simulink model "DinamicaCinematicaOrbital"  (R2024a)
settings: Solver=FixedStepAuto  StartTime=0.0  StopTime=tf  FixedStep=step_modelo  RelTol=1e-8  AbsTol=abs_tol
values from neighbouring files (symbols this model uses):
  J2 = 1082.63E-6    (= 0.00108263)    [constantes.m]
  mi = 3.9860044189*10^14    (= 398600441890000)    [constantes.m]
  omega_E = 7.29211585530*10^-5    (= 7.2921158553e-05)    [constantes.m]
  Re = 6378.1363*10^3    (= 6378136.3)    [constantes.m]
undefined symbols (not defined in the file or in its folder): a0_ini, Cd0, Cd1, drag, e0_ini, f0_ini, i0_ini, J2_dist, L0, L1, m0, m1, ohm0_ini, omega0_ini, pcoRad, r0, r0_dot_ini, t_man, theta0_ini, x0_dot, x0_dot_i, x0_dot_ini, x0_i, x0_ini, y0_dot_i, y0_dot_ini, y0_i, y0_ini, z0_dot_i, z0_dot_ini, z0_i, z0_ini
libraries: simulink x5
settings Model: PacingRate=500  Creator=rodri  LastModifiedBy=rodri
settings DataIOCC: SaveOutput=off  SaveTime=off
settings ModelReferenceCC: EnableRefExpFcnMdlSchedulingChecks=on
settings RTWCC: GPUComputeCapability=3.5

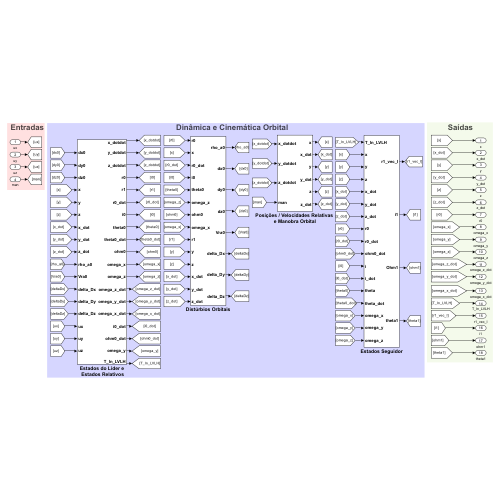
[thumbnail: Simulink's stored preview of the top-level diagram]
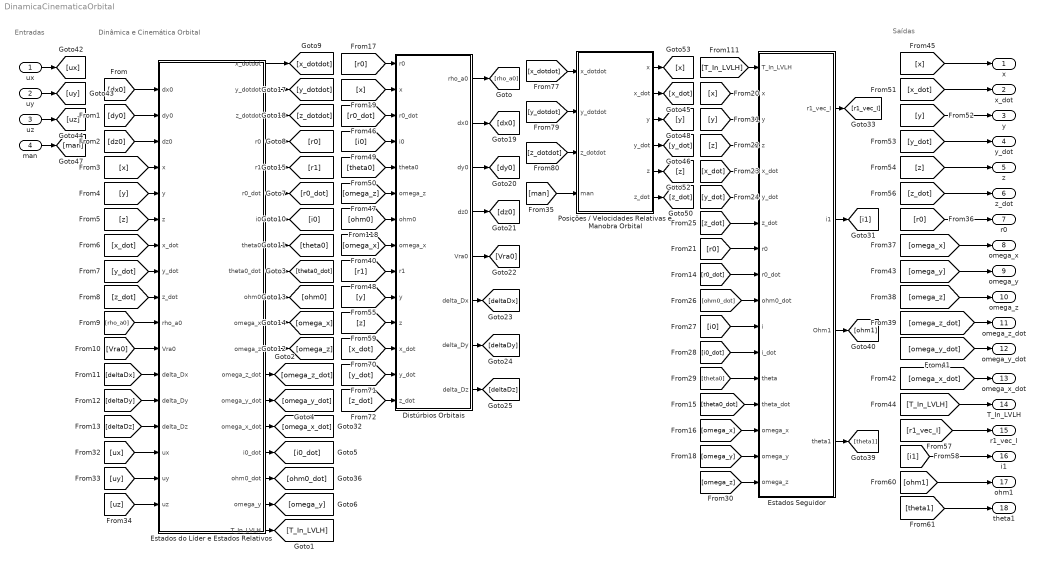
== system DinamicaCinematicaOrbital ==
  note: Saídas
  note: Dinâmica e Cinemática Orbital
  note: Entradas
  ux : Inport  OutDataTypeStr=double  PortDimensions=1
  uy : Inport  Port=2  OutDataTypeStr=double  PortDimensions=1
  uz : Inport  Port=3  OutDataTypeStr=double  PortDimensions=1
  man : Inport  Port=4  OutDataTypeStr=boolean
  Distúrbios Orbitais : Subsystem
  Estados Seguidor : Subsystem
  Estados do Líder e Estados Relativos : Subsystem
  Posições / Velocidades Relativas e Manobra Orbital : Subsystem
  x : Outport  OutDataTypeStr=double  PortDimensions=1  SampleTime=0
  x_dot : Outport  Port=2  OutDataTypeStr=double  PortDimensions=1  SampleTime=0
  y : Outport  Port=3  OutDataTypeStr=double  PortDimensions=1  SampleTime=0
  y_dot : Outport  Port=4  OutDataTypeStr=double  PortDimensions=1  SampleTime=0
  z : Outport  Port=5  OutDataTypeStr=double  PortDimensions=1  SampleTime=0
  z_dot : Outport  Port=6  OutDataTypeStr=double  PortDimensions=1  SampleTime=0
  r0 : Outport  Port=7  OutDataTypeStr=double  PortDimensions=1  SampleTime=0
  omega_x : Outport  Port=8  OutDataTypeStr=double  PortDimensions=1  SampleTime=0
  omega_y : Outport  Port=9
  omega_z : Outport  Port=10  OutDataTypeStr=double  PortDimensions=1  SampleTime=0
  omega_z_dot : Outport  Port=11  OutDataTypeStr=double  PortDimensions=1  SampleTime=0
  omega_y_dot : Outport  Port=12  OutDataTypeStr=double  PortDimensions=1  SampleTime=0
  omega_x_dot : Outport  Port=13  OutDataTypeStr=double  PortDimensions=1  SampleTime=0
  T_In_LVLH : Outport  Port=14
  r1_vec_I : Outport  Port=15
  i1 : Outport  Port=16
  ohm1 : Outport  Port=17
  theta1 : Outport  Port=18
  wires:
  Posições / Velocidades Relativas e Manobra Orbital/5(z) -> [z]
  Posições / Velocidades Relativas e Manobra Orbital/2(x_dot) -> [x_dot]
  Posições / Velocidades Relativas e Manobra Orbital/4(y_dot) -> [y_dot]
  Posições / Velocidades Relativas e Manobra Orbital/6(z_dot) -> [z_dot]
  Posições / Velocidades Relativas e Manobra Orbital/3(y) -> [y]
  Posições / Velocidades Relativas e Manobra Orbital/1(x) -> [x]
  Distúrbios Orbitais/1(rho_a0) -> [rho_a0]
  Estados do Líder e Estados Relativos/18(omega_y) -> [omega_y]
  Estados do Líder e Estados Relativos/14(omega_y_dot) -> [omega_y_dot]
  Estados do Líder e Estados Relativos/19(T_In_LVLH) -> [T_In_LVLH]
  Estados do Líder e Estados Relativos/13(omega_z_dot) -> [omega_z_dot]
  Estados do Líder e Estados Relativos/16(i0_dot) -> [i0_dot]
  Estados do Líder e Estados Relativos/12(omega_z) -> [omega_z]
  Estados do Líder e Estados Relativos/10(ohm0) -> [ohm0]
  Estados do Líder e Estados Relativos/2(y_dotdot) -> [y_dotdot]
  Estados do Líder e Estados Relativos/11(omega_x) -> [omega_x]
  Estados do Líder e Estados Relativos/4(r0) -> [r0]
  Estados do Líder e Estados Relativos/3(z_dotdot) -> [z_dotdot]
  Estados do Líder e Estados Relativos/6(r0_dot) -> [r0_dot]
  Estados do Líder e Estados Relativos/1(x_dotdot) -> [x_dotdot]
  Estados do Líder e Estados Relativos/8(theta0) -> [theta0]
  Estados do Líder e Estados Relativos/5(r1) -> [r1]
  Estados do Líder e Estados Relativos/7(i0) -> [i0]
  Estados do Líder e Estados Relativos/17(ohm0_dot) -> [ohm0_dot]
  Estados do Líder e Estados Relativos/15(omega_x_dot) -> [omega_x_dot]
  Estados do Líder e Estados Relativos/9(theta0_dot) -> [theta0_dot]
  [r1] -> Distúrbios Orbitais/9(r1)
  [i0] -> Distúrbios Orbitais/4(i0)
  [ohm0] -> Distúrbios Orbitais/7(ohm0)
  [x] -> Distúrbios Orbitais/2(x)
  [omega_z] -> Distúrbios Orbitais/6(omega_z)
  [r0_dot] -> Distúrbios Orbitais/3(r0_dot)
  [x_dot] -> Distúrbios Orbitais/12(x_dot)
  [r0] -> Distúrbios Orbitais/1(r0)
  [y] -> Distúrbios Orbitais/10(y)
  [z] -> Distúrbios Orbitais/11(z)
  [theta0] -> Distúrbios Orbitais/5(theta0)
  [z_dot] -> Distúrbios Orbitais/14(z_dot)
  [omega_x] -> Distúrbios Orbitais/8(omega_x)
  [y_dot] -> Distúrbios Orbitais/13(y_dot)
  [z_dotdot] -> Posições / Velocidades Relativas e Manobra Orbital/3(z_dotdot)
  [y_dotdot] -> Posições / Velocidades Relativas e Manobra Orbital/2(y_dotdot)
  [x_dotdot] -> Posições / Velocidades Relativas e Manobra Orbital/1(x_dotdot)
  Distúrbios Orbitais/2(dx0) -> [dx0]
  Distúrbios Orbitais/3(dy0) -> [dy0]
  Distúrbios Orbitais/4(dz0) -> [dz0]
  Distúrbios Orbitais/5(Vra0) -> [Vra0]
  Distúrbios Orbitais/6(delta_Dx) -> [deltaDx]
  Distúrbios Orbitais/7(delta_Dy) -> [deltaDy]
  Distúrbios Orbitais/8(delta_Dz) -> [deltaDz]
  [dx0] -> Estados do Líder e Estados Relativos/1(dx0)
  [dy0] -> Estados do Líder e Estados Relativos/2(dy0)
  [dz0] -> Estados do Líder e Estados Relativos/3(dz0)
  [x] -> Estados do Líder e Estados Relativos/4(x)
  [y] -> Estados do Líder e Estados Relativos/5(y)
  [z] -> Estados do Líder e Estados Relativos/6(z)
  [x_dot] -> Estados do Líder e Estados Relativos/7(x_dot)
  [y_dot] -> Estados do Líder e Estados Relativos/8(y_dot)
  [z_dot] -> Estados do Líder e Estados Relativos/9(z_dot)
  [rho_a0] -> Estados do Líder e Estados Relativos/10(rho_a0)
  [Vra0] -> Estados do Líder e Estados Relativos/11(Vra0)
  [deltaDx] -> Estados do Líder e Estados Relativos/12(delta_Dx)
  [deltaDz] -> Estados do Líder e Estados Relativos/14(delta_Dz)
  [deltaDy] -> Estados do Líder e Estados Relativos/13(delta_Dy)
  [x] -> Estados Seguidor/2(x)
  [i0] -> Estados Seguidor/11(i)
  Estados Seguidor/4(theta1) -> [theta1]
  Estados Seguidor/1(r1_vec_I) -> [r1_vec_I]
  [T_In_LVLH] -> Estados Seguidor/1(T_In_LVLH)
  [omega_z] -> Estados Seguidor/17(omega_z)
  [omega_x] -> Estados Seguidor/15(omega_x)
  [i0_dot] -> Estados Seguidor/12(i_dot)
  [ohm0_dot] -> Estados Seguidor/10(ohm0_dot)
  [theta0] -> Estados Seguidor/13(theta)
  [r0] -> Estados Seguidor/8(r0)
  Estados Seguidor/2(i1) -> [i1]
  [theta0_dot] -> Estados Seguidor/14(theta_dot)
  [z] -> Estados Seguidor/4(z)
  [z_dot] -> Estados Seguidor/7(z_dot)
  [y] -> Estados Seguidor/3(y)
  Estados Seguidor/3(Ohm1) -> [ohm1]
  [x_dot] -> Estados Seguidor/5(x_dot)
  [r0_dot] -> Estados Seguidor/9(r0_dot)
  [omega_y] -> Estados Seguidor/16(omega_y)
  [y_dot] -> Estados Seguidor/6(y_dot)
  ux/1 -> [ux]
  uy/1 -> [uy]
  uz/1 -> [uz]
  [ux] -> Estados do Líder e Estados Relativos/15(ux)
  [uy] -> Estados do Líder e Estados Relativos/16(uy)
  [uz] -> Estados do Líder e Estados Relativos/17(uz)
  man/1 -> [man]
  [man] -> Posições / Velocidades Relativas e Manobra Orbital/4(man)
  [r0] -> r0/1
  [omega_x] -> omega_x/1
  [omega_z] -> omega_z/1
  [omega_z_dot] -> omega_z_dot/1
  [omega_y_dot] -> omega_y_dot/1
  [omega_x_dot] -> omega_x_dot/1
  [omega_y] -> omega_y/1
  [T_In_LVLH] -> T_In_LVLH/1
  [x] -> x/1
  [x_dot] -> x_dot/1
  [y] -> y/1
  [y_dot] -> y_dot/1
  [z] -> z/1
  [z_dot] -> z_dot/1
  [r1_vec_I] -> r1_vec_I/1
  [i1] -> i1/1
  [ohm1] -> ohm1/1
  [theta1] -> theta1/1

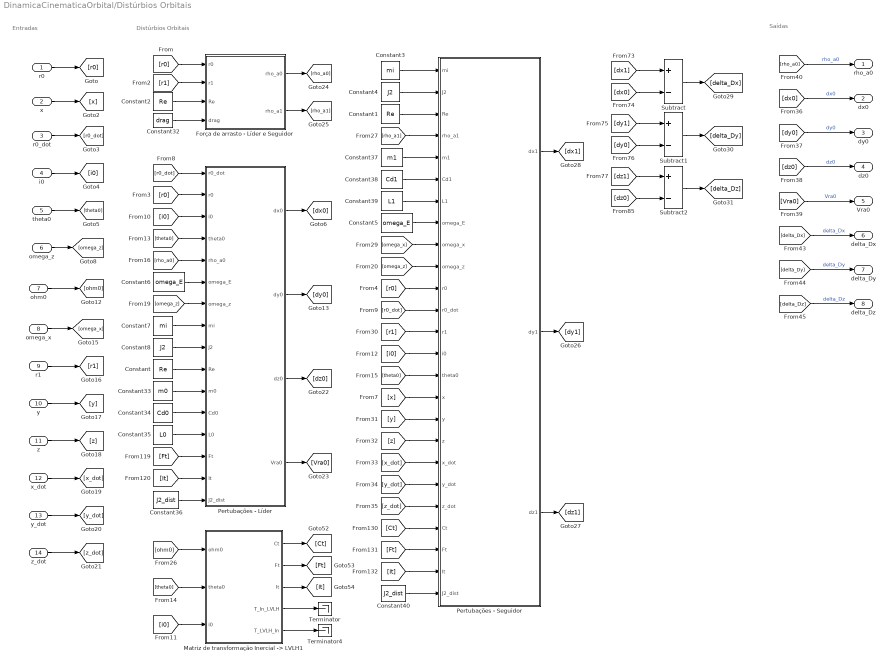
== system DinamicaCinematicaOrbital/Distúrbios Orbitais ==
  note: Distúrbios Orbitais
  note: Saídas
  note: Entradas
  r0 : Inport
  x : Inport  Port=2
  r0_dot : Inport  Port=3
  i0 : Inport  Port=4
  theta0 : Inport  Port=5
  omega_z : Inport  Port=6
  ohm0 : Inport  Port=7
  omega_x : Inport  Port=8
  r1 : Inport  Port=9
  y : Inport  Port=10
  z : Inport  Port=11
  x_dot : Inport  Port=12
  y_dot : Inport  Port=13
  z_dot : Inport  Port=14
  Constant : Constant  Value=Re
  Constant1 : Constant  Value=Re
  Constant2 : Constant  Value=Re
  Constant3 : Constant  Value=mi
  Constant32 : Constant  Value=drag  OutDataTypeStr=boolean
  Constant33 : Constant  Value=m0
  Constant34 : Constant  Value=Cd0
  Constant35 : Constant  Value=L0
  Constant36 : Constant  Value=J2_dist  OutDataTypeStr=boolean
  Constant37 : Constant  Value=m1
  Constant38 : Constant  Value=Cd1
  Constant39 : Constant  Value=L1
  Constant4 : Constant  Value=J2
  Constant40 : Constant  Value=J2_dist  OutDataTypeStr=boolean
  Constant5 : Constant  Value=omega_E
  Constant6 : Constant  Value=omega_E
  Constant7 : Constant  Value=mi
  Constant8 : Constant  Value=J2
  Força de arrasto - Líder e Seguidor : MATLAB Function  TreatAsAtomicUnit=on
  "Matriz de transformação Inercial -> LVLH1" : MATLAB Function  TreatAsAtomicUnit=on
  Pertubações - Líder : MATLAB Function  TreatAsAtomicUnit=on
  Pertubações - Seguidor : MATLAB Function  TreatAsAtomicUnit=on
  Subtract : Sum  Inputs=+-
  Subtract1 : Sum  Inputs=+-
  Subtract2 : Sum  Inputs=+-
  Terminator : Terminator
  Terminator4 : Terminator
  rho_a0 : Outport
  dx0 : Outport  Port=2
  dy0 : Outport  Port=3
  dz0 : Outport  Port=4
  Vra0 : Outport  Port=5
  delta_Dx : Outport  Port=6
  delta_Dy : Outport  Port=7
  delta_Dz : Outport  Port=8
  wires:
  Constant4/1 -> Pertubações - Seguidor/2(J2)
  Pertubações - Seguidor/3(dz1) -> [dz1]
  Constant6/1 -> Pertubações - Líder/6(omega_E)
  Subtract1/1 -> [delta_Dy]
  [dy0] -> dy0/1  "dy0"
  [omega_x] -> Pertubações - Seguidor/9(omega_x)
  [theta0] -> Pertubações - Seguidor/15(theta0)
  Subtract2/1 -> [delta_Dz]
  [It] -> Pertubações - Líder/15(It)
  "Matriz de transformação Inercial -> LVLH1"/5(T_LVLH_In) -> Terminator4/1
  [rho_a0] -> Pertubações - Líder/5(rho_a0)
  [y_dot] -> Pertubações - Seguidor/20(y_dot)
  [i0] -> Pertubações - Líder/3(i0)
  [z] -> Pertubações - Seguidor/18(z)
  Constant33/1 -> Pertubações - Líder/11(m0)
  Força de arrasto - Líder e Seguidor/2(rho_a1) -> [rho_a1]
  [x] -> Pertubações - Seguidor/16(x)
  "Matriz de transformação Inercial -> LVLH1"/4(T_In_LVLH) -> Terminator/1
  "Matriz de transformação Inercial -> LVLH1"/2(Ft) -> [Ft]
  [r0] -> Pertubações - Líder/2(r0)
  Constant3/1 -> Pertubações - Seguidor/1(mi)
  [y] -> Pertubações - Seguidor/17(y)
  Constant8/1 -> Pertubações - Líder/9(J2)
  [dy1] -> Subtract1/1
  Pertubações - Seguidor/2(dy1) -> [dy1]
  i0/1 -> [i0]
  [It] -> Pertubações - Seguidor/24(It)
  [rho_a1] -> Pertubações - Seguidor/4(rho_a1)
  "Matriz de transformação Inercial -> LVLH1"/3(It) -> [It]
  [rho_a0] -> rho_a0/1  "rho_a0"
  Constant/1 -> Pertubações - Líder/10(Re)
  [r0] -> Pertubações - Seguidor/11(r0)
  Constant38/1 -> Pertubações - Seguidor/6(Cd1)
  [Ft] -> Pertubações - Líder/14(Ft)
  [dy0] -> Subtract1/2
  Constant40/1 -> Pertubações - Seguidor/25(J2_dist)
  Constant1/1 -> Pertubações - Seguidor/3(Re)
  Constant7/1 -> Pertubações - Líder/8(mi)
  [r0] -> Força de arrasto - Líder e Seguidor/1(r0)
  "Matriz de transformação Inercial -> LVLH1"/1(Ct) -> [Ct]
  [dz1] -> Subtract2/1
  z_dot/1 -> [z_dot]
  [r1] -> Pertubações - Seguidor/13(r1)
  [z_dot] -> Pertubações - Seguidor/21(z_dot)
  [Ct] -> Pertubações - Seguidor/22(Ct)
  [dz0] -> Subtract2/2
  [r1] -> Força de arrasto - Líder e Seguidor/2(r1)
  [dx0] -> Subtract/2
  Constant5/1 -> Pertubações - Seguidor/8(omega_E)
  [i0] -> "Matriz de transformação Inercial -> LVLH1"/3(i0)
  [omega_z] -> Pertubações - Seguidor/10(omega_z)
  Constant34/1 -> Pertubações - Líder/12(Cd0)
  [theta0] -> "Matriz de transformação Inercial -> LVLH1"/2(theta0)
  Pertubações - Líder/3(dz0) -> [dz0]
  Constant36/1 -> Pertubações - Líder/16(J2_dist)
  [theta0] -> Pertubações - Líder/4(theta0)
  Pertubações - Líder/2(dy0) -> [dy0]
  [x_dot] -> Pertubações - Seguidor/19(x_dot)
  [r0_dot] -> Pertubações - Seguidor/12(r0_dot)
  Subtract/1 -> [delta_Dx]
  Constant2/1 -> Força de arrasto - Líder e Seguidor/3(Re)
  [i0] -> Pertubações - Seguidor/14(i0)
  [dx1] -> Subtract/1
  Constant39/1 -> Pertubações - Seguidor/7(L1)
  [r0_dot] -> Pertubações - Líder/1(r0_dot)
  [ohm0] -> "Matriz de transformação Inercial -> LVLH1"/1(ohm0)
  Pertubações - Líder/1(dx0) -> [dx0]
  [Ft] -> Pertubações - Seguidor/23(Ft)
  Constant32/1 -> Força de arrasto - Líder e Seguidor/4(drag)
  Constant35/1 -> Pertubações - Líder/13(L0)
  Força de arrasto - Líder e Seguidor/1(rho_a0) -> [rho_a0]
  Pertubações - Líder/4(Vra0) -> [Vra0]
  [delta_Dx] -> delta_Dx/1  "delta_Dx"
  Pertubações - Seguidor/1(dx1) -> [dx1]
  [omega_z] -> Pertubações - Líder/7(omega_z)
  Constant37/1 -> Pertubações - Seguidor/5(m1)
  r1/1 -> [r1]
  x_dot/1 -> [x_dot]
  [dz0] -> dz0/1  "dz0"
  [Vra0] -> Vra0/1  "Vra0"
  r0_dot/1 -> [r0_dot]
  z/1 -> [z]
  r0/1 -> [r0]
  [delta_Dz] -> delta_Dz/1  "delta_Dz"
  y_dot/1 -> [y_dot]
  y/1 -> [y]
  [dx0] -> dx0/1  "dx0"
  omega_z/1 -> [omega_z]
  x/1 -> [x]
  theta0/1 -> [theta0]
  omega_x/1 -> [omega_x]
  [delta_Dy] -> delta_Dy/1  "delta_Dy"
  ohm0/1 -> [ohm0]

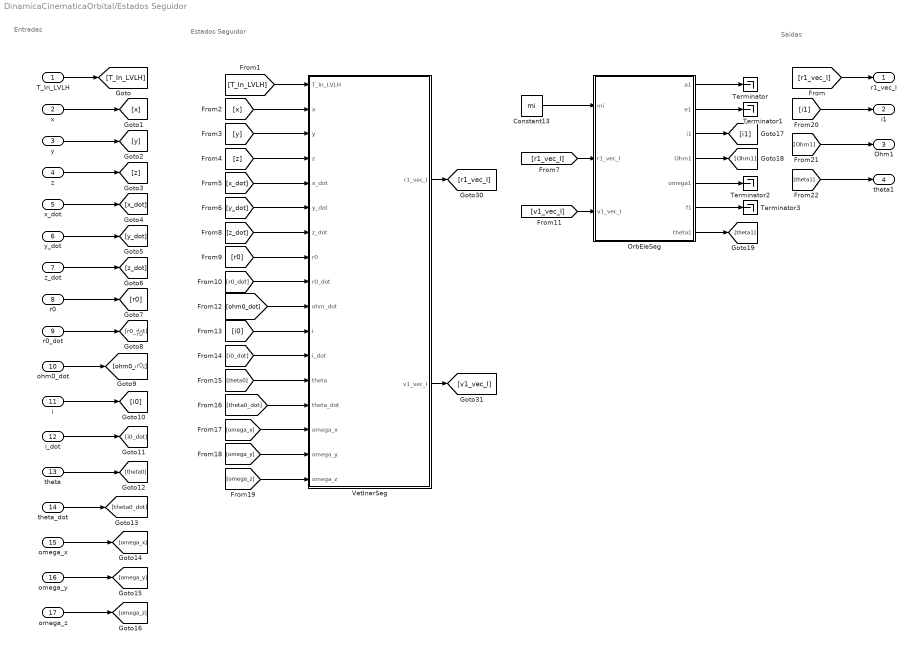
== system DinamicaCinematicaOrbital/Estados Seguidor ==
  note: r0
  note: Entradas
  note: Estados Seguidor
  note: Saídas
  note: r0
  T_In_LVLH : Inport
  x : Inport  Port=2
  y : Inport  Port=3
  z : Inport  Port=4
  x_dot : Inport  Port=5
  y_dot : Inport  Port=6
  z_dot : Inport  Port=7
  r0 : Inport  Port=8
  r0_dot : Inport  Port=9
  ohm0_dot : Inport  Port=10
  i : Inport  Port=11
  i_dot : Inport  Port=12
  theta : Inport  Port=13
  theta_dot : Inport  Port=14
  omega_x : Inport  Port=15
  omega_y : Inport  Port=16
  omega_z : Inport  Port=17
  Constant13 : Constant  Value=mi  SampleTime=-1
  OrbEleSeg : MATLAB Function  TreatAsAtomicUnit=on
  Terminator{,1..3} (4 alike) : Terminator
  VetInerSeg : MATLAB Function  TreatAsAtomicUnit=on
  r1_vec_I : Outport
  i1 : Outport  Port=2
  Ohm1 : Outport  Port=3
  theta1 : Outport  Port=4
  wires:
  VetInerSeg/2(v1_vec_I) -> [v1_vec_I]
  [r1_vec_I] -> OrbEleSeg/2(r1_vec_I)
  Constant13/1 -> OrbEleSeg/1(mi)
  [v1_vec_I] -> OrbEleSeg/3(v1_vec_I)
  VetInerSeg/1(r1_vec_I) -> [r1_vec_I]
  [r1_vec_I] -> r1_vec_I/1
  OrbEleSeg/1(a1) -> Terminator/1
  OrbEleSeg/2(e1) -> Terminator1/1
  OrbEleSeg/5(omega1) -> Terminator2/1
  OrbEleSeg/6(f1) -> Terminator3/1
  T_In_LVLH/1 -> [T_In_LVLH]
  x/1 -> [x]
  y/1 -> [y]
  z/1 -> [z]
  x_dot/1 -> [x_dot]
  y_dot/1 -> [y_dot]
  z_dot/1 -> [z_dot]
  r0/1 -> [r0]
  r0_dot/1 -> [r0_dot]
  ohm0_dot/1 -> [ohm0_dot]
  i/1 -> [i0]
  i_dot/1 -> [i0_dot]
  theta/1 -> [theta0]
  theta_dot/1 -> [theta0_dot]
  omega_x/1 -> [omega_x]
  omega_y/1 -> [omega_y]
  omega_z/1 -> [omega_z]
  [T_In_LVLH] -> VetInerSeg/1(T_In_LVLH)
  [x] -> VetInerSeg/2(x)
  [y] -> VetInerSeg/3(y)
  [z] -> VetInerSeg/4(z)
  [x_dot] -> VetInerSeg/5(x_dot)
  [y_dot] -> VetInerSeg/6(y_dot)
  [z_dot] -> VetInerSeg/7(z_dot)
  [r0] -> VetInerSeg/8(r0)
  [r0_dot] -> VetInerSeg/9(r0_dot)
  [ohm0_dot] -> VetInerSeg/10(ohm_dot)
  [i0] -> VetInerSeg/11(i)
  [i0_dot] -> VetInerSeg/12(i_dot)
  [theta0] -> VetInerSeg/13(theta)
  [theta0_dot] -> VetInerSeg/14(theta_dot)
  [omega_x] -> VetInerSeg/15(omega_x)
  [omega_y] -> VetInerSeg/16(omega_y)
  [omega_z] -> VetInerSeg/17(omega_z)
  [Ohm1] -> Ohm1/1
  [theta1] -> theta1/1
  [i1] -> i1/1
  OrbEleSeg/3(i1) -> [i1]
  OrbEleSeg/4(Ohm1) -> [Ohm1]
  OrbEleSeg/7(theta1) -> [theta1]

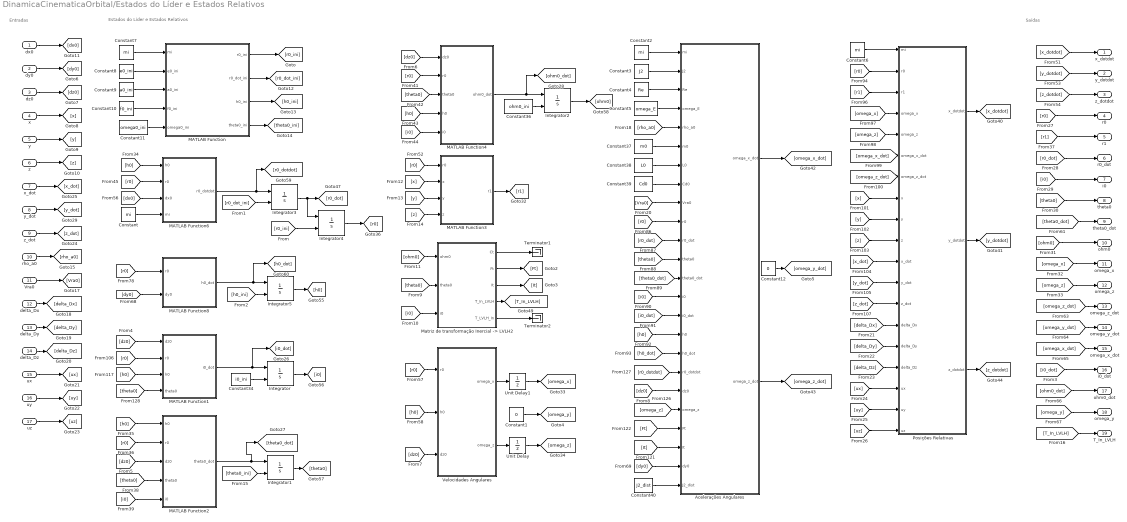
== system DinamicaCinematicaOrbital/Estados do Líder e Estados Relativos ==
  note: Entradas
  note: Saídas
  note: Estados do Líder e Estados Relativos
  dx0 : Inport
  dy0 : Inport  Port=2
  dz0 : Inport  Port=3
  x : Inport  Port=4
  y : Inport  Port=5
  z : Inport  Port=6
  x_dot : Inport  Port=7
  y_dot : Inport  Port=8
  z_dot : Inport  Port=9
  rho_a0 : Inport  Port=10
  Vra0 : Inport  Port=11
  delta_Dx : Inport  Port=12
  delta_Dy : Inport  Port=13
  delta_Dz : Inport  Port=14
  ux : Inport  Port=15
  uy : Inport  Port=16
  uz : Inport  Port=17
  Acelerações Angulares : MATLAB Function  TreatAsAtomicUnit=on
  Constant{,2,6..7} (4 alike) : Constant  Value=mi
  Constant1 : Constant  Value=0
  Constant10 : Constant  Value=f0_ini
  Constant11 : Constant  Value=omega0_ini
  Constant12 : Constant  Value=0
  Constant3 : Constant  Value=J2
  Constant34 : Constant  Value=i0_ini
  Constant36 : Constant  Value=ohm0_ini
  Constant37 : Constant  Value=m0
  Constant38 : Constant  Value=L0
  Constant39 : Constant  Value=Cd0
  Constant4 : Constant  Value=Re
  Constant40 : Constant  Value=J2_dist  OutDataTypeStr=boolean
  Constant5 : Constant  Value=omega_E
  Constant8 : Constant  Value=e0_ini
  Constant9 : Constant  Value=a0_ini
  Integrator : Integrator  InitialConditionSource=external  InitialCondition=i0_ini  AbsoluteTolerance=abs_tol
  Integrator1 : Integrator  InitialConditionSource=external  InitialCondition=theta0_ini  AbsoluteTolerance=abs_tol
  Integrator2 : Integrator  InitialConditionSource=external  InitialCondition=ohm0_ini  AbsoluteTolerance=abs_tol
  Integrator3 : Integrator  InitialConditionSource=external  InitialCondition=r0_dot_ini  AbsoluteTolerance=abs_tol
  Integrator4 : Integrator  InitialConditionSource=external  InitialCondition=r0  AbsoluteTolerance=abs_tol
  Integrator5 : Integrator  InitialConditionSource=external  InitialCondition=i0_ini  AbsoluteTolerance=abs_tol
  MATLAB Function : MATLAB Function  TreatAsAtomicUnit=on
  MATLAB Function1 : MATLAB Function  TreatAsAtomicUnit=on
  MATLAB Function2 : MATLAB Function  TreatAsAtomicUnit=on
  MATLAB Function3 : MATLAB Function  TreatAsAtomicUnit=on
  MATLAB Function4 : MATLAB Function  TreatAsAtomicUnit=on
  MATLAB Function6 : MATLAB Function  TreatAsAtomicUnit=on
  MATLAB Function8 : MATLAB Function  TreatAsAtomicUnit=on
  "Matriz de transformação Inercial -> LVLH2" : MATLAB Function  TreatAsAtomicUnit=on
  Posições Relativas : MATLAB Function  TreatAsAtomicUnit=on
  Terminator1 : Terminator
  Terminator2 : Terminator
  Unit Delay : UnitDelay  SampleTime=-1  HasFrameUpgradeWarning=on
  Unit Delay1 : UnitDelay  SampleTime=-1  HasFrameUpgradeWarning=on
  Velocidades Angulares : MATLAB Function  TreatAsAtomicUnit=on
  x_dotdot : Outport
  y_dotdot : Outport  Port=2
  z_dotdot : Outport  Port=3
  r0 : Outport  Port=4
  r1 : Outport  Port=5
  r0_dot : Outport  Port=6
  i0 : Outport  Port=7
  theta0 : Outport  Port=8
  theta0_dot : Outport  Port=9
  ohm0 : Outport  Port=10
  omega_x : Outport  Port=11
  omega_z : Outport  Port=12
  omega_z_dot : Outport  Port=13
  omega_y_dot : Outport  Port=14
  omega_x_dot : Outport  Port=15
  i0_dot : Outport  Port=16
  ohm0_dot : Outport  Port=17
  omega_y : Outport  Port=18
  T_In_LVLH : Outport  Port=19
  wires:
  [h0] -> Acelerações Angulares/16(h0)
  [theta0_dot] -> Acelerações Angulares/13(theta0_dot)
  "Matriz de transformação Inercial -> LVLH2"/5(T_LVLH_In) -> Terminator2/1
  Constant2/1 -> Acelerações Angulares/1(mi)
  [dz0] -> MATLAB Function2/3(dz0)
  [y] -> Posições Relativas/9(y)
  [Vra0] -> Acelerações Angulares/9(Vra0)
  "Matriz de transformação Inercial -> LVLH2"/4(T_In_LVLH) -> [T_In_LVLH]
  [Ft] -> Acelerações Angulares/21(Ft)
  [r0] -> MATLAB Function8/1(r0)
  [r0_ini] -> Integrator4/2
  [i0] -> MATLAB Function2/5(i0)
  [omega_z_dot] -> Posições Relativas/7(omega_z_dot)
  Constant3/1 -> Acelerações Angulares/2(J2)
  [i0] -> Acelerações Angulares/14(i0)
  [h0_ini] -> Integrator5/2
  Velocidades Angulares/2(omega_z) -> Unit Delay/1
  [theta0] -> MATLAB Function2/4(theta0)
  [dz0] -> Acelerações Angulares/19(dz0)
  z/1 -> [z]
  dy0/1 -> [dy0]
  [r0] -> Posições Relativas/2(r0)
  Posições Relativas/2(y_dotdot) -> [y_dotdot]
  [r0_dotdot] -> Acelerações Angulares/18(r0_dotdot)
  [dz0] -> MATLAB Function1/1(dz0)
  MATLAB Function2/1(theta0_dot) -> Integrator1/1, [theta0_dot]
  [delta_Dz] -> Posições Relativas/16(delta_Dz)
  [i0] -> MATLAB Function4/5(i0)
  [r0] -> MATLAB Function2/2(r0)
  [r0] -> r0/1
  MATLAB Function/4(theta0_ini) -> [theta0_ini]
  Integrator1/1 -> [theta0]
  Constant36/1 -> Integrator2/2
  [ux] -> Posições Relativas/17(ux)
  [dy0] -> MATLAB Function8/2(dy0)
  [h0_dot] -> Acelerações Angulares/17(h0_dot)
  [r0] -> MATLAB Function4/2(r0)
  MATLAB Function8/1(h0_dot) -> Integrator5/1, [h0_dot]
  [x] -> MATLAB Function3/2(x)
  Integrator2/1 -> [ohm0]
  MATLAB Function6/1(r0_dotdot) -> Integrator3/1, [r0_dotdot]
  [h0] -> MATLAB Function1/3(h0)
  Constant34/1 -> Integrator/2
  [theta0] -> MATLAB Function1/4(theta0)
  Constant12/1 -> [omega_y_dot]
  MATLAB Function1/1(i0_dot) -> [i0_dot], Integrator/1
  [dz0] -> Velocidades Angulares/3(dz0)
  [r0] -> MATLAB Function1/2(r0)
  Integrator5/1 -> [h0]
  [x_dot] -> Posições Relativas/11(x_dot)
  z_dot/1 -> [z_dot]
  Integrator4/1 -> [r0]
  [y] -> MATLAB Function3/3(y)
  Constant40/1 -> Acelerações Angulares/24(J2_dist)
  [delta_Dy] -> Posições Relativas/15(delta_Dy)
  [r0_dot] -> Acelerações Angulares/11(r0_dot)
  Posições Relativas/1(x_dotdot) -> [x_dotdot]
  MATLAB Function4/1(ohm0_dot) -> Integrator2/1, [ohm0_dot]
  [It] -> Acelerações Angulares/22(It)
  [r0] -> MATLAB Function6/2(r0)
  Constant39/1 -> Acelerações Angulares/8(Cd0)
  [dz0] -> MATLAB Function4/1(dz0)
  [r0] -> MATLAB Function3/1(r0)
  Constant1/1 -> [omega_y]
  [r0_dot] -> r0_dot/1
  Constant38/1 -> Acelerações Angulares/7(L0)
  [omega_y_dot] -> omega_y_dot/1
  Constant6/1 -> Posições Relativas/1(mi)
  [r0] -> Velocidades Angulares/1(r0)
  "Matriz de transformação Inercial -> LVLH2"/3(It) -> [It]
  [r0] -> Acelerações Angulares/10(r0)
  delta_Dx/1 -> [delta_Dx]
  [omega_x_dot] -> Posições Relativas/6(omega_x_dot)
  [uz] -> Posições Relativas/19(uz)
  [dy0] -> Acelerações Angulares/23(dy0)
  "Matriz de transformação Inercial -> LVLH2"/2(Ft) -> [Ft]
  [ohm0] -> "Matriz de transformação Inercial -> LVLH2"/1(ohm0)
  [omega_z] -> omega_z/1
  Integrator/1 -> [i0]
  [i0_dot] -> Acelerações Angulares/15(i0_dot)
  Integrator3/1 -> [r0_dot], Integrator4/1
  MATLAB Function/3(h0_ini) -> [h0_ini]
  [omega_x] -> Posições Relativas/4(omega_x)
  [rho_a0] -> Acelerações Angulares/5(rho_a0)
  [h0] -> Velocidades Angulares/2(h0)
  Constant/1 -> MATLAB Function6/4(mi)
  [y_dot] -> Posições Relativas/12(y_dot)
  [h0] -> MATLAB Function2/1(h0)
  [x_dotdot] -> x_dotdot/1
  [i0] -> "Matriz de transformação Inercial -> LVLH2"/3(i0)
  [omega_z] -> Posições Relativas/5(omega_z)
  [r1] -> Posições Relativas/3(r1)
  Constant37/1 -> Acelerações Angulares/6(m0)
  Constant5/1 -> Acelerações Angulares/4(omega_E)
  Acelerações Angulares/1(omega_x_dot) -> [omega_x_dot]
  [dx0] -> MATLAB Function6/3(dx0)
  Velocidades Angulares/1(omega_x) -> Unit Delay1/1
  [r0_dot_ini] -> Integrator3/2
  [theta0_ini] -> Integrator1/2
  [theta0] -> Acelerações Angulares/12(theta0)
  [z_dot] -> Posições Relativas/13(z_dot)
  [z] -> Posições Relativas/10(z)
  [x] -> Posições Relativas/8(x)
  Constant4/1 -> Acelerações Angulares/3(Re)
  [theta0] -> MATLAB Function4/3(theta0)
  Constant7/1 -> MATLAB Function/1(mi)
  [uy] -> Posições Relativas/18(uy)
  MATLAB Function/2(r0_dot_ini) -> [r0_dot_ini]
  [delta_Dx] -> Posições Relativas/14(delta_Dx)
  delta_Dz/1 -> [delta_Dz]
  Constant8/1 -> MATLAB Function/2(e0_ini)
  [z] -> MATLAB Function3/4(z)
  Constant9/1 -> MATLAB Function/3(a0_ini)
  [theta0] -> "Matriz de transformação Inercial -> LVLH2"/2(theta0)
  [h0] -> MATLAB Function6/1(h0)
  Acelerações Angulares/2(omega_z_dot) -> [omega_z_dot]
  "Matriz de transformação Inercial -> LVLH2"/1(Ct) -> Terminator1/1
  MATLAB Function3/1(r1) -> [r1]
  Constant10/1 -> MATLAB Function/4(f0_ini)
  [omega_z] -> Acelerações Angulares/20(omega_z)
  MATLAB Function/1(r0_ini) -> [r0_ini]
  Constant11/1 -> MATLAB Function/5(omega0_ini)
  [h0] -> MATLAB Function4/4(h0)
  Posições Relativas/3(z_dotdot) -> [z_dotdot]
  y_dot/1 -> [y_dot]
  delta_Dy/1 -> [delta_Dy]
  [z_dotdot] -> z_dotdot/1
  y/1 -> [y]
  rho_a0/1 -> [rho_a0]
  [i0] -> i0/1
  Vra0/1 -> [Vra0]
  [omega_z_dot] -> omega_z_dot/1
  uz/1 -> [uz]
  [omega_y] -> omega_y/1
  ux/1 -> [ux]
  [ohm0] -> ohm0/1
  [omega_x_dot] -> omega_x_dot/1
  x/1 -> [x]
  [r1] -> r1/1
  [y_dotdot] -> y_dotdot/1
  x_dot/1 -> [x_dot]
  [i0_dot] -> i0_dot/1
  dz0/1 -> [dz0]
  [ohm0_dot] -> ohm0_dot/1
  [theta0_dot] -> theta0_dot/1
  [omega_x] -> omega_x/1
  dx0/1 -> [dx0]
  [theta0] -> theta0/1
  [T_In_LVLH] -> T_In_LVLH/1
  uy/1 -> [uy]
  Unit Delay/1 -> [omega_z]
  Unit Delay1/1 -> [omega_x]

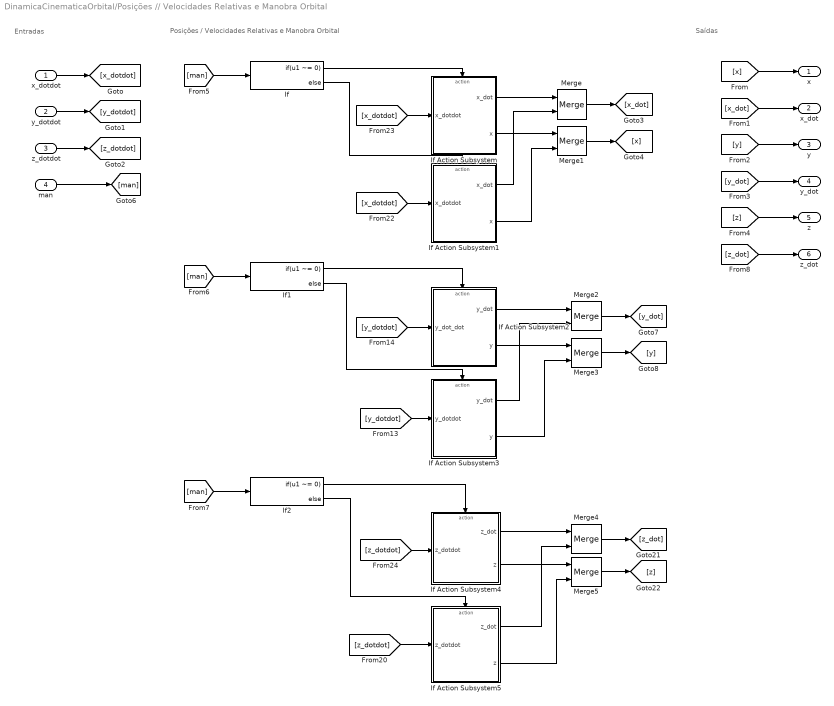
== system DinamicaCinematicaOrbital/Posições // Velocidades Relativas e Manobra Orbital ==
  note: Posições / Velocidades Relativas e Manobra Orbital
  note: Entradas
  note: Saídas
  x_dotdot : Inport
  y_dotdot : Inport  Port=2
  z_dotdot : Inport  Port=3
  man : Inport  Port=4
  If : If  IfExpression=u1 ~= 0
  If Action Subsystem : Subsystem  TreatAsAtomicUnit=on
  If Action Subsystem1 : Subsystem  TreatAsAtomicUnit=on
  If Action Subsystem2 : Subsystem  TreatAsAtomicUnit=on
  If Action Subsystem3 : Subsystem  TreatAsAtomicUnit=on
  If Action Subsystem4 : Subsystem  TreatAsAtomicUnit=on
  If Action Subsystem5 : Subsystem  TreatAsAtomicUnit=on
  If1 : If  IfExpression=u1 ~= 0
  If2 : If  IfExpression=u1 ~= 0
  Merge : Merge  InitialOutput=x0_dot_ini
  Merge1 : Merge  InitialOutput=x0_ini
  Merge2 : Merge  InitialOutput=y0_dot_ini
  Merge3 : Merge  InitialOutput=y0_ini
  Merge4 : Merge  InitialOutput=z0_dot_ini
  Merge5 : Merge  InitialOutput=z0_ini
  x : Outport
  x_dot : Outport  Port=2
  y : Outport  Port=3
  y_dot : Outport  Port=4
  z : Outport  Port=5
  z_dot : Outport  Port=6
  wires:
  [y_dotdot] -> If Action Subsystem2/1(y_dot_dot)
  Merge/1 -> [x_dot]
  If Action Subsystem4/2(z) -> Merge5/1
  [x] -> x/1
  If2/2 -> If Action Subsystem5/Action
  If Action Subsystem/2(x) -> Merge1/1
  [z_dotdot] -> If Action Subsystem5/1(z_dotdot)
  [z_dot] -> z_dot/1
  man/1 -> [man]
  If1/2 -> If Action Subsystem3/Action
  If1/1 -> If Action Subsystem2/Action
  [y_dotdot] -> If Action Subsystem3/1(y_dotdot)
  [man] -> If2/1
  If Action Subsystem3/1(y_dot) -> Merge2/2
  Merge2/1 -> [y_dot]
  If2/1 -> If Action Subsystem4/Action
  If Action Subsystem1/1(x_dot) -> Merge/2
  [man] -> If1/1
  Merge3/1 -> [y]
  Merge1/1 -> [x]
  If Action Subsystem2/1(y_dot) -> Merge2/1
  If Action Subsystem4/1(z_dot) -> Merge4/1
  Merge4/1 -> [z_dot]
  [x_dotdot] -> If Action Subsystem1/1(x_dotdot)
  If Action Subsystem/1(x_dot) -> Merge/1
  [z_dotdot] -> If Action Subsystem4/1(z_dotdot)
  If Action Subsystem2/2(y) -> Merge3/1
  If Action Subsystem1/2(x) -> Merge1/2
  If Action Subsystem3/2(y) -> Merge3/2
  If/1 -> If Action Subsystem/Action
  [man] -> If/1
  If/2 -> If Action Subsystem1/Action
  [x_dot] -> x_dot/1
  If Action Subsystem5/1(z_dot) -> Merge4/2
  y_dotdot/1 -> [y_dotdot]
  If Action Subsystem5/2(z) -> Merge5/2
  [x_dotdot] -> If Action Subsystem/1(x_dotdot)
  [z] -> z/1
  x_dotdot/1 -> [x_dotdot]
  z_dotdot/1 -> [z_dotdot]
  [y] -> y/1
  [y_dot] -> y_dot/1
  Merge5/1 -> [z]

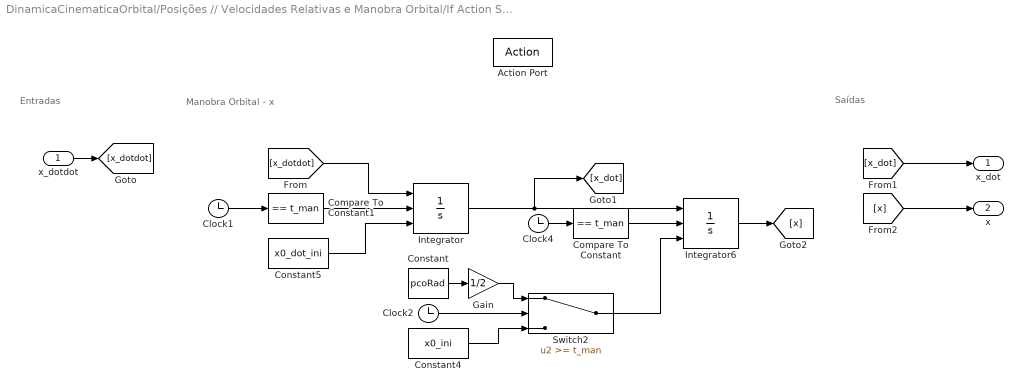
== system DinamicaCinematicaOrbital/Posições // Velocidades Relativas e Manobra Orbital/If Action Subsystem ==
  note: Entradas
  note: Manobra Orbital - x
  note: Saídas
  x_dotdot : Inport
  Action Port : ActionPort  ActionPortLabel=if(u1 ~= 0)
  Clock1 : Clock
  Clock2 : Clock
  Clock4 : Clock
  Compare To Constant : simulink/Logic and Bit Operations/Compare To Constant  relop===  const=t_man  OutDataTypeStr=boolean
  Compare To Constant1 : simulink/Logic and Bit Operations/Compare To Constant  relop===  const=t_man  OutDataTypeStr=boolean
  Constant : Constant  Value=pcoRad
  Constant4 : Constant  Value=x0_ini  SampleTime=-1
  Constant5 : Constant  Value=x0_dot_ini  SampleTime=-1
  Gain : Gain  Gain=1/2
  Integrator : Integrator  ExternalReset=either  InitialConditionSource=external  InitialCondition=x0_dot  AbsoluteTolerance=abs_tol
  Integrator6 : Integrator  ExternalReset=either  InitialConditionSource=external  InitialCondition=x0_dot  AbsoluteTolerance=abs_tol
  Switch2 : Switch  Threshold=t_man  SaturateOnIntegerOverflow=off  InputSameDT=off
  x_dot : Outport  InitialOutput=x0_dot_ini
  x : Outport  Port=2  InitialOutput=x0_ini
  wires:
  Switch2/1 -> Integrator6/3
  Compare To Constant/1 -> Integrator6/2
  Compare To Constant1/1 -> Integrator/2
  Clock2/1 -> Switch2/2
  Constant4/1 -> Switch2/3
  Clock4/1 -> Compare To Constant/1
  Clock1/1 -> Compare To Constant1/1
  Constant/1 -> Gain/1
  Integrator/1 -> [x_dot], Integrator6/1
  Gain/1 -> Switch2/1
  Constant5/1 -> Integrator/3
  x_dotdot/1 -> [x_dotdot]
  [x_dotdot] -> Integrator/1
  Integrator6/1 -> [x]
  [x_dot] -> x_dot/1
  [x] -> x/1

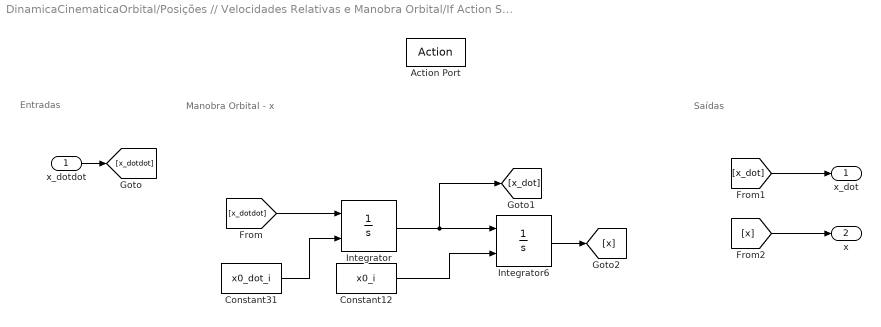
== system DinamicaCinematicaOrbital/Posições // Velocidades Relativas e Manobra Orbital/If Action Subsystem1 ==
  note: Manobra Orbital - x
  note: Entradas
  note: Saídas
  x_dotdot : Inport
  Action Port : ActionPort  ActionPortLabel=else
  Constant12 : Constant  Value=x0_i  SampleTime=-1
  Constant31 : Constant  Value=x0_dot_i  SampleTime=-1
  Integrator : Integrator  InitialConditionSource=external  InitialCondition=x0_dot  AbsoluteTolerance=abs_tol
  Integrator6 : Integrator  InitialConditionSource=external  InitialCondition=x0_dot  AbsoluteTolerance=abs_tol
  x_dot : Outport  InitialOutput=x0_dot_ini
  x : Outport  Port=2  InitialOutput=x0_ini
  wires:
  Integrator/1 -> [x_dot], Integrator6/1
  Constant31/1 -> Integrator/2
  Constant12/1 -> Integrator6/2
  x_dotdot/1 -> [x_dotdot]
  [x_dotdot] -> Integrator/1
  Integrator6/1 -> [x]
  [x_dot] -> x_dot/1
  [x] -> x/1

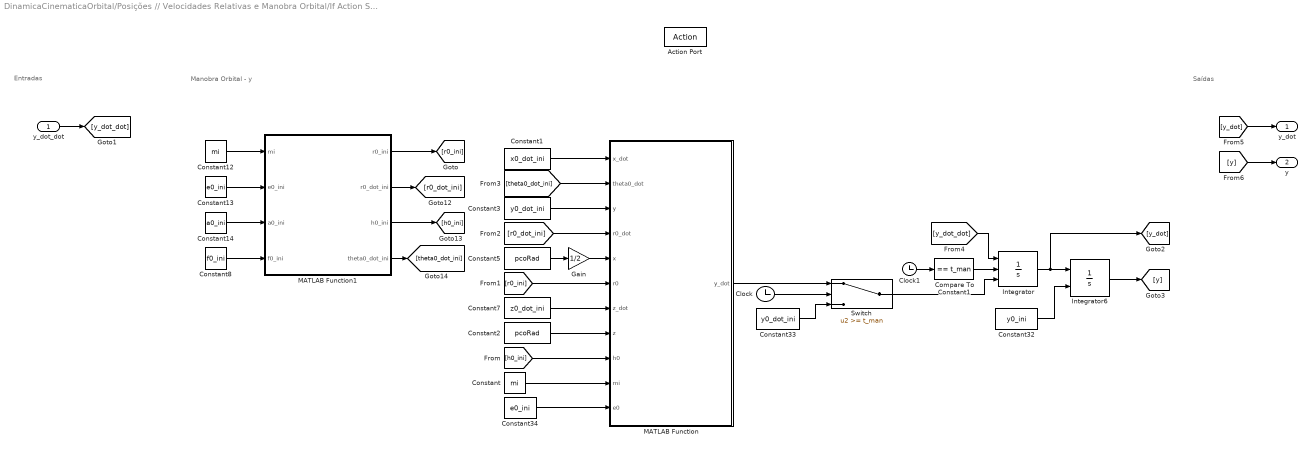
== system DinamicaCinematicaOrbital/Posições // Velocidades Relativas e Manobra Orbital/If Action Subsystem2 ==
  note: Entradas
  note: Saídas
  note: Manobra Orbital - y
  y_dot_dot : Inport
  Action Port : ActionPort  ActionPortLabel=if(u1 ~= 0)
  Clock : Clock
  Clock1 : Clock
  Compare To Constant1 : simulink/Logic and Bit Operations/Compare To Constant  relop===  const=t_man  OutDataTypeStr=boolean
  Constant : Constant  Value=mi  SampleTime=-1
  Constant1 : Constant  Value=x0_dot_ini
  Constant12 : Constant  Value=mi
  Constant13 : Constant  Value=e0_ini
  Constant14 : Constant  Value=a0_ini
  Constant2 : Constant  Value=pcoRad
  Constant3 : Constant  Value=y0_dot_ini
  Constant32 : Constant  Value=y0_ini  SampleTime=-1
  Constant33 : Constant  Value=y0_dot_ini  SampleTime=-1
  Constant34 : Constant  Value=e0_ini  SampleTime=-1  LockScale=on
  Constant5 : Constant  Value=pcoRad
  Constant7 : Constant  Value=z0_dot_ini
  Constant8 : Constant  Value=f0_ini
  Gain : Gain  Gain=1/2
  Integrator : Integrator  ExternalReset=either  InitialConditionSource=external  InitialCondition=x0_dot  AbsoluteTolerance=abs_tol
  Integrator6 : Integrator  InitialConditionSource=external  InitialCondition=x0_dot  AbsoluteTolerance=abs_tol
  MATLAB Function : MATLAB Function  TreatAsAtomicUnit=on
  MATLAB Function1 : MATLAB Function  TreatAsAtomicUnit=on
  Switch : Switch  Threshold=t_man  SaturateOnIntegerOverflow=off  InputSameDT=off
  y_dot : Outport  InitialOutput=y0_dot_ini
  y : Outport  Port=2  InitialOutput=y0_ini
  wires:
  Switch/1 -> Integrator/3
  Clock/1 -> Switch/2
  Constant32/1 -> Integrator6/2
  Constant33/1 -> Switch/3
  Compare To Constant1/1 -> Integrator/2
  MATLAB Function/1(y_dot) -> Switch/1
  Clock1/1 -> Compare To Constant1/1
  Constant/1 -> MATLAB Function/10(mi)
  Constant34/1 -> MATLAB Function/11(e0)
  Integrator6/1 -> [y]
  [h0_ini] -> MATLAB Function/9(h0)
  Constant2/1 -> MATLAB Function/8(z)
  Constant7/1 -> MATLAB Function/7(z_dot)
  [r0_ini] -> MATLAB Function/6(r0)
  Gain/1 -> MATLAB Function/5(x)
  [r0_dot_ini] -> MATLAB Function/4(r0_dot)
  Constant3/1 -> MATLAB Function/3(y)
  [theta0_dot_ini] -> MATLAB Function/2(theta0_dot)
  Constant1/1 -> MATLAB Function/1(x_dot)
  Integrator/1 -> Integrator6/1, [y_dot]
  Constant5/1 -> Gain/1
  Constant8/1 -> MATLAB Function1/4(f0_ini)
  MATLAB Function1/1(r0_ini) -> [r0_ini]
  MATLAB Function1/3(h0_ini) -> [h0_ini]
  Constant14/1 -> MATLAB Function1/3(a0_ini)
  MATLAB Function1/2(r0_dot_ini) -> [r0_dot_ini]
  Constant12/1 -> MATLAB Function1/1(mi)
  Constant13/1 -> MATLAB Function1/2(e0_ini)
  MATLAB Function1/4(theta0_dot_ini) -> [theta0_dot_ini]
  y_dot_dot/1 -> [y_dot_dot]
  [y_dot_dot] -> Integrator/1
  [y_dot] -> y_dot/1
  [y] -> y/1

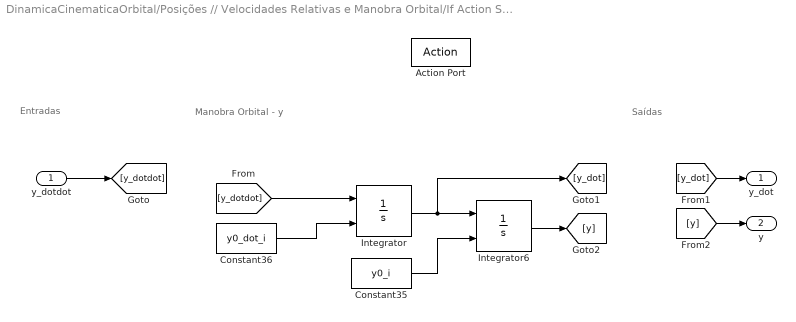
== system DinamicaCinematicaOrbital/Posições // Velocidades Relativas e Manobra Orbital/If Action Subsystem3 ==
  note: Entradas
  note: Saídas
  note: Manobra Orbital - y
  y_dotdot : Inport
  Action Port : ActionPort  ActionPortLabel=else
  Constant35 : Constant  Value=y0_i  SampleTime=-1
  Constant36 : Constant  Value=y0_dot_i  SampleTime=-1
  Integrator : Integrator  InitialConditionSource=external  InitialCondition=x0_dot  AbsoluteTolerance=abs_tol
  Integrator6 : Integrator  InitialConditionSource=external  InitialCondition=x0_dot  AbsoluteTolerance=abs_tol
  y_dot : Outport  InitialOutput=y0_dot_ini
  y : Outport  Port=2  InitialOutput=y0_ini
  wires:
  Integrator6/1 -> [y]
  Integrator/1 -> Integrator6/1, [y_dot]
  Constant36/1 -> Integrator/2
  Constant35/1 -> Integrator6/2
  y_dotdot/1 -> [y_dotdot]
  [y_dotdot] -> Integrator/1
  [y] -> y/1
  [y_dot] -> y_dot/1

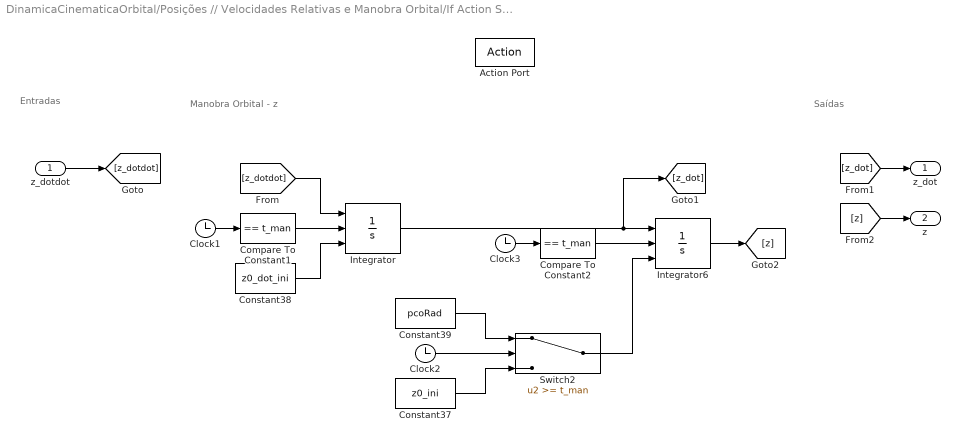
== system DinamicaCinematicaOrbital/Posições // Velocidades Relativas e Manobra Orbital/If Action Subsystem4 ==
  note: Entradas
  note: Saídas
  note: Manobra Orbital - z
  z_dotdot : Inport
  Action Port : ActionPort  ActionPortLabel=if(u1 ~= 0)
  Clock1 : Clock
  Clock2 : Clock
  Clock3 : Clock
  Compare To Constant1 : simulink/Logic and Bit Operations/Compare To Constant  relop===  const=t_man  OutDataTypeStr=boolean
  Compare To Constant2 : simulink/Logic and Bit Operations/Compare To Constant  relop===  const=t_man  OutDataTypeStr=boolean
  Constant37 : Constant  Value=z0_ini  SampleTime=-1
  Constant38 : Constant  Value=z0_dot_ini  SampleTime=-1
  Constant39 : Constant  Value=pcoRad  SampleTime=-1
  Integrator : Integrator  ExternalReset=either  InitialConditionSource=external  InitialCondition=x0_dot  AbsoluteTolerance=abs_tol
  Integrator6 : Integrator  ExternalReset=either  InitialConditionSource=external  InitialCondition=x0_dot  AbsoluteTolerance=abs_tol
  Switch2 : Switch  Threshold=t_man  SaturateOnIntegerOverflow=off  InputSameDT=off
  z_dot : Outport  InitialOutput=z0_dot_ini
  z : Outport  Port=2  InitialOutput=z0_ini
  wires:
  Integrator6/1 -> [z]
  Switch2/1 -> Integrator6/3
  Compare To Constant2/1 -> Integrator6/2
  Compare To Constant1/1 -> Integrator/2
  Clock2/1 -> Switch2/2
  Clock1/1 -> Compare To Constant1/1
  Clock3/1 -> Compare To Constant2/1
  Integrator/1 -> [z_dot], Integrator6/1
  Constant39/1 -> Switch2/1
  Constant37/1 -> Switch2/3
  Constant38/1 -> Integrator/3
  z_dotdot/1 -> [z_dotdot]
  [z_dotdot] -> Integrator/1
  [z_dot] -> z_dot/1
  [z] -> z/1

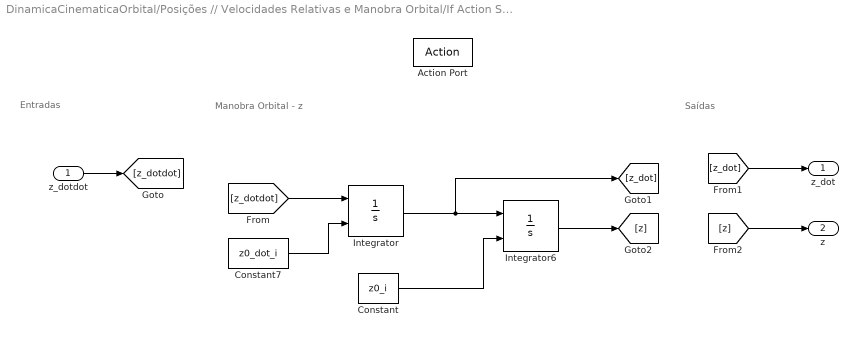
== system DinamicaCinematicaOrbital/Posições // Velocidades Relativas e Manobra Orbital/If Action Subsystem5 ==
  note: Entradas
  note: Saídas
  note: Manobra Orbital - z
  z_dotdot : Inport
  Action Port : ActionPort  ActionPortLabel=else
  Constant : Constant  Value=z0_i  SampleTime=-1
  Constant7 : Constant  Value=z0_dot_i  SampleTime=-1
  Integrator : Integrator  InitialConditionSource=external  InitialCondition=x0_dot  AbsoluteTolerance=abs_tol
  Integrator6 : Integrator  InitialConditionSource=external  InitialCondition=x0_dot  AbsoluteTolerance=abs_tol
  z_dot : Outport  InitialOutput=z0_dot_ini
  z : Outport  Port=2  InitialOutput=z0_ini
  wires:
  Integrator6/1 -> [z]
  Integrator/1 -> Integrator6/1, [z_dot]
  Constant7/1 -> Integrator/2
  Constant/1 -> Integrator6/2
  z_dotdot/1 -> [z_dotdot]
  [z_dotdot] -> Integrator/1
  [z_dot] -> z_dot/1
  [z] -> z/1

== matlab function DinamicaCinematicaOrbital/Estados do Líder e Estados Relativos/MATLAB Function ==
  data: mi input; r0_ini output; e0_ini input; a0_ini input; f0_ini input; r0_dot_ini output; h0_ini output; omega0_ini input; theta0_ini output
function [r0_ini,r0_dot_ini,h0_ini,theta0_ini] = fcn(mi,e0_ini,a0_ini,f0_ini,omega0_ini)

r0_ini = a0_ini*(1 - e0_ini^2)/(1 + e0_ini*cos(f0_ini));
r0_dot_ini = e0_ini*sin(f0_ini)*sqrt(mi/(a0_ini*(1 - e0_ini^2)));
h0_ini = sqrt(-(e0_ini^2 - 1)*mi*a0_ini);
theta0_ini = omega0_ini + f0_ini;

== matlab function DinamicaCinematicaOrbital/Estados Seguidor/OrbEleSeg ==
  data: mi input; a1 output; r1_vec_I input; e1 output; i1 output; Ohm1 output; omega1 output; f1 output; theta1 output; v1_vec_I input
function [a1,e1,i1,Ohm1,omega1,f1,theta1] = fcn(mi,r1_vec_I,v1_vec_I)



[a1,e1,i1,Ohm1,omega1,f1,theta1,~] = orb_elem(mi,r1_vec_I',v1_vec_I');

== matlab function DinamicaCinematicaOrbital/Estados Seguidor/VetInerSeg ==
  data: T_In_LVLH input; r1_vec_I output; x input; y input; z input; x_dot input; y_dot input; z_dot input; r0 input; r0_dot input; v1_vec_I output; ohm_dot input; i input; i_dot input; theta input; theta_dot input; omega_x input; omega_y input; omega_z input
function [r1_vec_I,v1_vec_I] = fcn(T_In_LVLH,x,y,z,x_dot,y_dot,z_dot,r0,r0_dot,ohm_dot,i,i_dot,theta,theta_dot,omega_x,omega_y,omega_z)

%% Elementos da matrix
A = T_In_LVLH(1,1);
B = T_In_LVLH(1,2);
E = T_In_LVLH(1,3);
C = T_In_LVLH(2,1);
D = T_In_LVLH(2,2);
F = T_In_LVLH(2,3);
G = T_In_LVLH(3,1);
H = T_In_LVLH(3,2);
K = T_In_LVLH(3,3);

%% Componentes da posição
rs = r0;

rho_x = A*x + C*y + G*z;
rho_y = B*x + D*y + H*z;
rho_z = E*x + F*y + K*z;

Xsl = A*rs + rho_x;
Ysl = B*rs + rho_y;
Zsl = E*rs + rho_z;

%% Componentes da velocidade
X0_dot = r0_dot*T_In_LVLH(1,1) + r0*(-T_In_LVLH(1,2))*ohm_dot + r0*T_In_LVLH(3,1)*sin(theta)*i_dot + r0*T_In_LVLH(2,1)*theta_dot;
Y0_dot = r0_dot*T_In_LVLH(1,2) + r0*T_In_LVLH(1,1)*ohm_dot - r0*(-T_In_LVLH(3,1))*sin(theta)*i_dot + r0*T_In_LVLH(2,2)*theta_dot;
Z0_dot = r0_dot*T_In_LVLH(1,3) + r0*cos(i)*sin(theta)*i_dot + r0*T_In_LVLH(2,3)*theta_dot;

xi_dot = A*x_dot + C*y_dot + G*z_dot;
yi_dot = B*x_dot + D*y_dot + H*z_dot;
zi_dot = E*x_dot + F*y_dot + K*z_dot;

omega_I = T_In_LVLH'*[omega_x;omega_y;omega_z];
rho_I = [rho_x rho_y rho_z];
rot = cross(omega_I',rho_I);

Xsl_dot = X0_dot + xi_dot + rot(1);
Ysl_dot = Y0_dot + yi_dot + rot(2);
Zsl_dot = Z0_dot + zi_dot + rot(3);

%% Vetores inerciais finais
r1_vec_I = [Xsl Ysl Zsl]';
v1_vec_I = [Xsl_dot Ysl_dot Zsl_dot]';

%% Elementos orbitais calculados

% r_sl = sqrt(Xsl^2 + Ysl^2 + Zsl^2);
% 
% epsilon_sl = (1/2)*(Xsl_dot^2 + Ysl_dot^2 + Zsl_dot^2) - mi*(Xsl^2 + Ysl^2 + Zsl^2)^(-1/2);
% 
% a_sl = -mi/(2*epsilon_sl);
% 
% h_sl = sqrt((Ysl*Zsl_dot - Zsl*Ysl_dot)^2 + (Xsl*Zsl_dot - Zsl*Xsl_dot)^2 + (Xsl*Ysl_dot - Ysl*Xsl_dot)^2);
% 
% i_sl = acos((Xsl*Ysl_dot - Ysl*Xsl_dot)/h_sl);
% 
% theta_sl = asin(Zsl/(r_sl*sin(i_sl)));
% 
% e_sl = (1 - (h_sl^2)/(mi*a_sl))^(1/2);
% 
% f_sl = acos((1/e_sl)*((h_sl^2)/(mi*r_sl) - 1));
% 
% omega_sl = theta_sl - acos((1/e_sl)*(h_sl^2/(mi*r_sl) - 1));
% 
% theta_sl2 = f_sl + omega_sl;
% 
% ohm_sl = atan((Ysl*Zsl_dot - Zsl*Ysl_dot)/(Xsl*Zsl_dot - Zsl*Xsl_dot));

== matlab function DinamicaCinematicaOrbital/Distúrbios Orbitais/Pertubações - Seguidor ==
  data: mi input; dx1 output; J2 input; Re input; rho_a1 input; m1 input; Cd1 input; L1 input; omega_E input; omega_x input; omega_z input; r0 input; r0_dot input; r1 input; i0 input; theta0 input; x input; y input; z input; x_dot input; y_dot input; z_dot input; dy1 output; dz1 output; Ct input; Ft input; It input; J2_dist input
function [dx1,dy1,dz1] = fcn(mi,J2,Re,rho_a1,m1,Cd1,L1,omega_E,omega_x,omega_z,r0,r0_dot,r1,i0,theta0,x,y,z,x_dot,y_dot,z_dot,Ct,Ft,It,J2_dist)

b1 = m1/(Cd1*((L1^2)*sqrt(2)));

if J2_dist == false
    j2 = 0;
else
    j2 = J2;
end


k2 = (r0 + x)*sin(i0)*sin(theta0) + y*cos(theta0)*sin(i0) + z*cos(i0);
k1 = (5*k2^2)/(r1^2) - 1;
k3 = (r0_dot + x_dot - omega_z*y) - (Ft*omega_E*z - y*It*omega_E);
k4 = (r0*omega_z + y_dot + omega_z*x - omega_x*z) - ((r0 + x)*It*omega_E - z*Ct*omega_E);
k5 = (z_dot + omega_x*y) - (y*Ct*omega_E - (r0 + x)*Ft*omega_E);

Vra1 = sqrt(k3^2 + k4^2 + k5^2);
dx1 = ((3*mi*j2*Re^2)/(2*(r1^5)))*(k1*(r0 + x) - 2*k2*sin(i0)*sin(theta0)) - (1/2)*(rho_a1/b1)*Vra1*k3*10^-2; %24
dy1 = ((3*mi*j2*Re^2)/(2*(r1^5)))*(k1*y - 2*k2*sin(i0)*cos(theta0)) - (1/2)*(rho_a1/b1)*Vra1*k4*10^-2; %25
dz1 = ((3*mi*j2*Re^2)/(2*(r1^5)))*(k1*z - 2*k2*cos(i0)) - (1/2)*(rho_a1/b1)*Vra1*k5*10^-2; %26

== matlab function DinamicaCinematicaOrbital/Estados do Líder e Estados Relativos/Velocidades Angulares ==
  data: r0 input; omega_x output; h0 input; dz0 input; omega_z output
function [omega_x,omega_z] = fcn(r0,h0,dz0)

omega_x = dz0*r0/h0;
omega_z = h0/(r0^2);

== matlab function DinamicaCinematicaOrbital/Estados do Líder e Estados Relativos/Acelerações Angulares ==
  data: mi input; omega_x_dot output; J2 input; Re input; omega_E input; rho_a0 input; m0 input; L0 input; Cd0 input; Vra0 input; r0 input; r0_dot input; theta0 input; theta0_dot input; i0 input; i0_dot input; h0 input; h0_dot input; omega_z_dot output; r0_dotdot input; dz0 input; omega_z input; Ft input; It input; dy0 input; J2_dist input
function [omega_x_dot,omega_z_dot] = fcn(mi,J2,Re,omega_E,rho_a0,m0,L0,Cd0,Vra0,r0,r0_dot,theta0,theta0_dot,i0,i0_dot,h0,h0_dot,r0_dotdot,dz0,omega_z,Ft,It,dy0,J2_dist)

b0  = m0/(Cd0*(L0^2));

if J2_dist == false
    J2 = 0;
end

% omega_z_dot = (h0_dot*r0^2 - h0*2*r0*r0_dot)/(r0^4);
% omega_z_dot = (-2*h0/(r0^3))*(-mi/(r0^2) + h0^2/(r0^3));
omega_z_dot = dy0/r0 - 2*(h0/r0^3)*r0_dot;


dj2z0_dot = ((-3*mi*J2*Re^2)/2)*(((theta0_dot*cos(theta0)*sin(2*i0) + sin(theta0)*2*i0_dot*cos(2*i0))*(r0^4) - sin(theta0)*sin(2*i0)*4*r0*r0_dot)/(r0^8));

Ft_dot = theta0_dot*(-sin(theta0))*sin(i0) + cos(theta0)*i0_dot*cos(i0);
It_dot = i0_dot*(-sin(i0));
Vra0_dot = (1/2)*((r0_dot^2 + (r0*omega_z - It*omega_E*r0)^2 + (Ft*omega_E*r0)^2 )^(-1/2))*(2*r0_dot*r0_dotdot + 2*(r0*omega_z - It*omega_E*r0)*((r0_dot*omega_z + r0*omega_z_dot) - omega_E*(It_dot*r0 + It*r0_dot)) + 2*(Ft*omega_E*r0)*(omega_E*(Ft_dot*r0 + Ft*r0_dot)));
daz0_dot = (-rho_a0*omega_E/(2*b0))*(Vra0_dot*Ft*r0 + Vra0*(Ft_dot*r0 + Ft*r0_dot));

dz0_dot = dj2z0_dot + daz0_dot;

%omega_x_dot = ((dz0_dot*r0 + dz0*r0_dot)*h0 - (dz0*r0*h0_dot))/(h0^2);
omega_x_dot = -((dz0*dy0*r0^2)/(h0^2)) + ((dz0*r0_dot)/(h0)) + ((r0*dz0_dot)/(h0));

== matlab function DinamicaCinematicaOrbital/Distúrbios Orbitais/Força de arrasto - Líder e Seguidor ==
  data: r0 input; r1 input; rho_a0 output; rho_a1 output; Re input; drag input
function [rho_a0,rho_a1] = fcn(r0,r1,Re,drag)

if drag == false
    rho_a0 = 0;
    rho_a1 = 0;
else
    rho_a0 = densAtm(r0-Re);
    rho_a1 = densAtm(r1-Re);
end

== matlab function DinamicaCinematicaOrbital/Estados do Líder e Estados Relativos/MATLAB Function6 ==
  data: h0 input; r0_dotdot output; r0 input; dx0 input; mi input
function r0_dotdot = fcn(h0,r0,dx0,mi)

r0_dotdot = (h0^2)/(r0^3) - mi/(r0^2) + dx0;

== matlab function DinamicaCinematicaOrbital/Estados do Líder e Estados Relativos/MATLAB Function8 ==
  data: r0 input; h0_dot output; dy0 input
function h0_dot   = fcn(r0,dy0)

h0_dot = dy0*r0;

== matlab function DinamicaCinematicaOrbital/Estados do Líder e Estados Relativos/MATLAB Function1 ==
  data: dz0 input; i0_dot output; r0 input; h0 input; theta0 input
function i0_dot = fcn(dz0,r0,h0,theta0)

i0_dot = (dz0*r0/h0)*cos(theta0);

== matlab function DinamicaCinematicaOrbital/Estados do Líder e Estados Relativos/MATLAB Function2 ==
  data: h0 input; theta0_dot output; r0 input; dz0 input; theta0 input; i0 input
function theta0_dot = fcn(h0,r0,dz0,theta0,i0)

if i0 == 0
    theta0_dot = h0/(r0^2);
else
    theta0_dot = h0/(r0^2)-((dz0*r0*sin(theta0))/(h0*sin(i0)))*cos(i0);
end

== matlab function DinamicaCinematicaOrbital/Estados do Líder e Estados Relativos/MATLAB Function4 ==
  data: dz0 input; ohm0_dot output; r0 input; theta0 input; h0 input; i0 input
function ohm0_dot = fcn(dz0,r0,theta0,h0,i0)

if i0 == 0
    ohm0_dot = 0;
else
    ohm0_dot = (dz0*r0*sin(theta0))/(h0*sin(i0));
end

== matlab function DinamicaCinematicaOrbital/Estados do Líder e Estados Relativos/MATLAB Function3 ==
  data: r0 input; r1 output; x input; y input; z input
function r1 = fcn(r0,x,y,z)

r1 = sqrt((r0+x)^2 + y^2 + z^2);

== matlab function DinamicaCinematicaOrbital/Distúrbios Orbitais/Matriz de transformação Inercial -> LVLH1 ==
  data: ohm0 input; Ct output; Ft output; theta0 input; i0 input; It output; T_In_LVLH output; T_LVLH_In output
function [Ct,Ft,It,T_In_LVLH,T_LVLH_In] = fcn(ohm0,theta0,i0)

[T_In_LVLH,T_LVLH_In] = TransInerLVLH(ohm0,theta0,i0);

Ct = T_In_LVLH(1,3);
Ft = T_In_LVLH(2,3);
It = T_In_LVLH(3,3);

== matlab function DinamicaCinematicaOrbital/Estados do Líder e Estados Relativos/Posições Relativas ==
  data: mi input; x_dotdot output; r0 input; r1 input; omega_x input; omega_z input; omega_x_dot input; omega_z_dot input; x input; y input; z input; x_dot input; y_dot input; z_dot input; delta_Dx input; delta_Dy input; delta_Dz input; y_dotdot output; z_dotdot output; ux input; uy input; uz input
function [x_dotdot,y_dotdot,z_dotdot] = fcn(mi,r0,r1,omega_x,omega_z,omega_x_dot,omega_z_dot,x,y,z,x_dot,y_dot,z_dot,delta_Dx,delta_Dy,delta_Dz,ux,uy,uz)

x_dotdot = omega_z_dot*y + 2*omega_z*y_dot + omega_z*(omega_z*x - omega_x*z) - (mi/(r1^3))*(r0 + x) + (mi/(r0^2)) + delta_Dx + ux; %13
y_dotdot = (omega_x^2)*y + 2*omega_x*z_dot + (omega_z^2)*y - 2*omega_z*x_dot - omega_z_dot*x + omega_x_dot*z - (mi/(r1^3))*y + delta_Dy + uy; %13
z_dotdot = -omega_x_dot*y - 2*omega_x*y_dot - omega_x*(omega_z*x - omega_x*z) - (mi/(r1^3))*z + delta_Dz + uz; %13

== matlab function DinamicaCinematicaOrbital/Estados do Líder e Estados Relativos/Matriz de transformação Inercial -> LVLH2 ==
  data: ohm0 input; Ct output; Ft output; theta0 input; i0 input; It output; T_In_LVLH output; T_LVLH_In output
function [Ct,Ft,It,T_In_LVLH,T_LVLH_In] = fcn(ohm0,theta0,i0)

[T_In_LVLH,T_LVLH_In] = TransInerLVLH(ohm0,theta0,i0);

Ct = T_In_LVLH(1,3);
Ft = T_In_LVLH(2,3);
It = T_In_LVLH(3,3);

== matlab function DinamicaCinematicaOrbital/Posições // Velocidades Relativas e Manobra Orbital/If Action Subsystem2/MATLAB Function ==
  data: x_dot input; y_dot output; theta0_dot input; y input; r0_dot input; x input; r0 input; z_dot input; z input; h0 input; mi input; e0 input
function y_dot = fcn(x_dot,theta0_dot,y,r0_dot,x,r0,z_dot,z,h0,mi,e0)

a0 = (h0^2/mi)/(1 - e0^2);

if ((r0+x)^2+y^2+z^2) < 0
    A1 = 0;
else
    A1 = mi/(sqrt((r0+x)^2+y^2+z^2))-mi/(2*a0);
end

A2 = (x_dot-theta0_dot*y+r0_dot)^2-z_dot^2;

if (2*A1-A2) < 0
    A1 = 0;
    A2 = 0;
end

A3 = theta0_dot*(x+r0);

y_dot = sqrt(2*A1-A2)-A3;

== matlab function DinamicaCinematicaOrbital/Posições // Velocidades Relativas e Manobra Orbital/If Action Subsystem2/MATLAB Function1 ==
  data: mi input; r0_ini output; e0_ini input; a0_ini input; f0_ini input; r0_dot_ini output; h0_ini output; theta0_dot_ini output
function [r0_ini,r0_dot_ini,h0_ini,theta0_dot_ini] = fcn(mi,e0_ini,a0_ini,f0_ini)

r0_ini = a0_ini*(1 - e0_ini^2)/(1 + e0_ini*cos(f0_ini));
r0_dot_ini = e0_ini*sin(f0_ini)*sqrt(mi/(a0_ini*(1 - e0_ini^2)));
h0_ini = sqrt(-(e0_ini^2 - 1)*mi*a0_ini);
theta0_dot_ini = h0_ini/r0_ini^2;

== matlab function DinamicaCinematicaOrbital/Distúrbios Orbitais/Pertubações - Líder ==
  data: r0_dot input; dx0 output; r0 input; i0 input; theta0 input; rho_a0 input; dy0 output; dz0 output; omega_E input; omega_z input; mi input; J2 input; Re input; m0 input; Cd0 input; L0 input; Vra0 output; Ft input; It input; J2_dist input
function [dx0,dy0,dz0,Vra0] = fcn(r0_dot,r0,i0,theta0,rho_a0,omega_E,omega_z,mi,J2,Re,m0,Cd0,L0,Ft,It,J2_dist)

b0 = m0/(Cd0*(L0^2));

Vra0 = sqrt((r0_dot)^2 + (r0*omega_z - It*omega_E*r0)^2 + (Ft*omega_E*r0)^2);

if J2_dist == false
    j2 = 0;
else
    j2 = J2;
end

dx0 = ((-3*mi*j2*Re^2)/(2*r0^4))*(1 - 3*(sin(i0)^2)*(sin(theta0)^2)) - (1/2)*(rho_a0/b0)*Vra0*r0_dot*10^-2;
dy0 = ((-3*mi*j2*Re^2)/(2*r0^4))*((sin(i0)^2)*(sin(2*theta0))) - (1/2)*(rho_a0/b0)*Vra0*(r0*omega_z - It*omega_E*r0)*10^-2;
dz0 = ((-3*mi*j2*Re^2)/(2*r0^4))*(sin(theta0)*(sin(2*i0))) - (1/2)*(rho_a0/b0)*Vra0*Ft*omega_E*r0*10^-2;
